simulink model "check_serial_2msg_processor_2"  (R2021a)
settings: Solver=FixedStepDiscrete  StartTime=0.0  StopTime=inf  FixedStep=time_step  RelTol=1e-3
model workspace (MAT data in the model file):
  time_step = 0.01
undefined symbols (not defined in the file or in its folder): DiscIntNeverNeededParam, Serial_Port, Standard_Devices
libraries: sldrtlib x6
settings Model: OrderedModelArguments=off  Creator=Rahul Subramanian  LastModifiedBy=Rahul Subramanian
settings SolverCC: AlgebraicLoopSolver=TrustRegion
settings DebuggingCC: SFMachineParentedDataDiag=warning
settings RTWCC: Description=Simulink Desktop Real-Time  SystemTargetFile=sldrt.tlc  TemplateMakefile=sldrt.tmf  RTWCompilerOptimization=on
settings CodeAppCC: MaxIdLength=95
settings SimulinkDesktopRealTimeCC: TargetPreCompLibLocation=C:\Program Files\MATLAB\R2021a\toolbox\sldrt\lib\win64

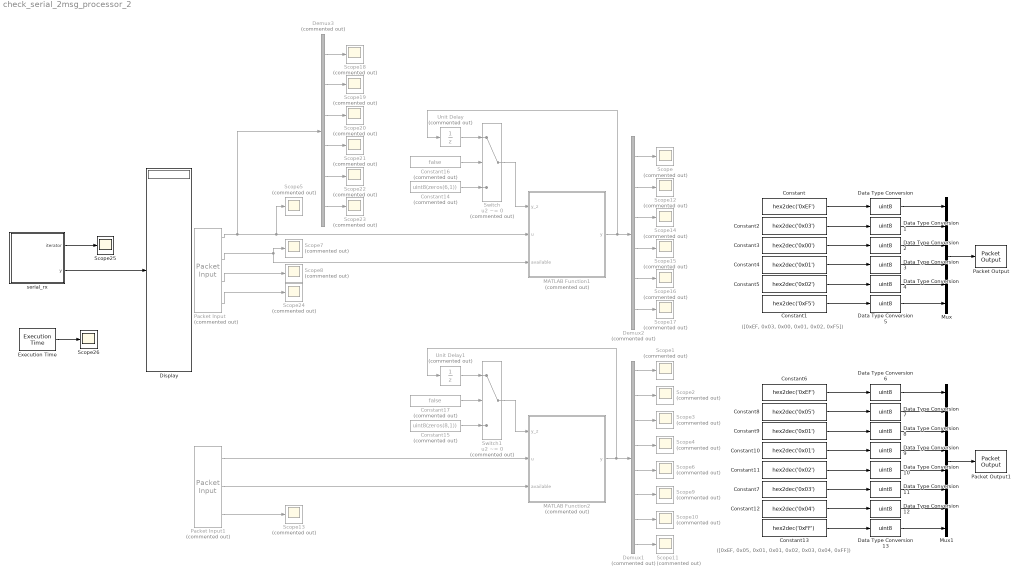
== system check_serial_2msg_processor_2 ==
  note: ([0xEF, 0x05, 0x01, 0x01, 0x02, 0x03, 0x04, 0xFF])
  note: ([0xEF, 0x03, 0x00, 0x01, 0x02, 0xF5])
  Constant : Constant  Value=hex2dec('0xEF')
  Constant1 : Constant  Value=hex2dec('0xF5')
  Constant10 : Constant  Value=hex2dec('0x01')
  Constant11 : Constant  Value=hex2dec('0x02')
  Constant12 : Constant  Value=hex2dec('0x04')
  Constant13 : Constant  Value=hex2dec('0xFF')
  Constant14 : Constant  Commented=on  Value=uint8(zeros(6,1))
  Constant15 : Constant  Commented=on  Value=uint8(zeros(8,1))
  Constant16 : Constant  Commented=on  Value=false
  Constant17 : Constant  Commented=on  Value=false
  Constant2 : Constant  Value=hex2dec('0x03')
  Constant3 : Constant  Value=hex2dec('0x00')
  Constant4 : Constant  Value=hex2dec('0x01')
  Constant5 : Constant  Value=hex2dec('0x02')
  Constant6 : Constant  Value=hex2dec('0xEF')
  Constant7 : Constant  Value=hex2dec('0x03')
  Constant8 : Constant  Value=hex2dec('0x05')
  Constant9 : Constant  Value=hex2dec('0x01')
  Data Type Conversion{,1..13} (14 alike) : DataTypeConversion  OutDataTypeStr=uint8
  Demux1 : Demux  Commented=on  Outputs=8
  Demux2 : Demux  Commented=on  Outputs=6
  Demux3 : Demux  Commented=on  Outputs=6
  Display : Display
  Execution Time : sldrtlib/Target Profiling/Execution Time  ShowTaskTimes=off
      settings: SourceProductBaseCode=WT
  MATLAB Function1 : MATLAB Function  Commented=on  TreatAsAtomicUnit=on
  MATLAB Function2 : MATLAB Function  Commented=on  TreatAsAtomicUnit=on
  Mux : Mux  Inputs=6
  Mux1 : Mux  Inputs=8
  Packet Input : sldrtlib/Packet Input  Commented=on  SampleTime=time_step  MaxMissedTicks=inf  ShowMissedTicks=on  YieldWhenWaiting=off  DrvName=Standard_Devices/Serial_Port  DrvAddress=5  DrvOptions=[115200 8 0 0 0 0 0 0]  PacketSize=6  DataTypes='6*uint8'  ShowReady=on  ShowError=on  PacketID=1  ByteOrder=1  ShowTimestamp=off
      settings: AttributesFormatString=Serial Port [5]
  Packet Input1 : sldrtlib/Packet Input  Commented=on  SampleTime=time_step  MaxMissedTicks=inf  ShowMissedTicks=on  YieldWhenWaiting=off  DrvName=Standard_Devices/Serial_Port  DrvAddress=5  DrvOptions=[115200 8 0 0 0 0 0 0]  PacketSize=8  DataTypes='8*uint8'  ShowReady=on  ShowError=off  PacketID=1  ByteOrder=1  ShowTimestamp=off
      settings: AttributesFormatString=Serial Port [5]
  Packet Output : sldrtlib/Packet Output  SampleTime=time_step  MaxMissedTicks=inf  ShowMissedTicks=off  YieldWhenWaiting=off  DrvName=Standard_Devices/Serial_Port  DrvAddress=5  DrvOptions=[115200 8 0 0 0 0 0 0]  PacketSize=6  DataTypes='6*uint8'  ShowReady=off  ShowError=off  PacketID=1  ByteOrder=1  InitialValue=[]  FinalValue=[]
      settings: AttributesFormatString=Serial Port [5]
  Packet Output1 : sldrtlib/Packet Output  SampleTime=time_step  MaxMissedTicks=inf  ShowMissedTicks=off  YieldWhenWaiting=off  DrvName=Standard_Devices/Serial_Port  DrvAddress=5  DrvOptions=[115200 8 0 0 0 0 0 0]  PacketSize=8  DataTypes='8*uint8'  ShowReady=off  ShowError=off  PacketID=1  ByteOrder=1  InitialValue=[]  FinalValue=[]
      settings: AttributesFormatString=Serial Port [5]
  Scope{,1..24} (25 alike) : Scope  Commented=on
  Scope25 : Scope
  Scope26 : Scope
  Switch : Switch  Commented=on  Criteria=u2 ~= 0
  Switch1 : Switch  Commented=on  Criteria=u2 ~= 0
  Unit Delay : UnitDelay  Commented=on  SampleTime=-1  HasFrameUpgradeWarning=on
  Unit Delay1 : UnitDelay  Commented=on  SampleTime=-1  HasFrameUpgradeWarning=on
  serial_rx : Subsystem
  wires:
  Constant/1 -> Data Type Conversion/1
  Constant2/1 -> Data Type Conversion1/1
  Constant3/1 -> Data Type Conversion2/1
  Constant4/1 -> Data Type Conversion3/1
  Constant5/1 -> Data Type Conversion4/1
  Data Type Conversion/1 -> Mux/1
  Data Type Conversion1/1 -> Mux/2
  Data Type Conversion2/1 -> Mux/3
  Data Type Conversion3/1 -> Mux/4
  Data Type Conversion4/1 -> Mux/5
  Packet Input/3 -> Scope8/1
  Mux/1 -> Packet Output/1
  Constant1/1 -> Data Type Conversion5/1
  Data Type Conversion5/1 -> Mux/6
  Data Type Conversion11/1 -> Mux1/6
  Constant7/1 -> Data Type Conversion11/1
  Mux1/1 -> Packet Output1/1
  Data Type Conversion10/1 -> Mux1/5
  Data Type Conversion9/1 -> Mux1/4
  Data Type Conversion8/1 -> Mux1/3
  Data Type Conversion7/1 -> Mux1/2
  Data Type Conversion6/1 -> Mux1/1
  Constant11/1 -> Data Type Conversion10/1
  Constant10/1 -> Data Type Conversion9/1
  Constant9/1 -> Data Type Conversion8/1
  Constant8/1 -> Data Type Conversion7/1
  Constant6/1 -> Data Type Conversion6/1
  Data Type Conversion12/1 -> Mux1/7
  Data Type Conversion13/1 -> Mux1/8
  Constant12/1 -> Data Type Conversion12/1
  Constant13/1 -> Data Type Conversion13/1
  Demux2/1 -> Scope/1
  MATLAB Function1/1(y) -> Unit Delay/1, Demux2/1
  Demux2/2 -> Scope12/1
  Demux2/3 -> Scope14/1
  Demux2/4 -> Scope15/1
  Demux2/5 -> Scope16/1
  Demux2/6 -> Scope17/1
  Switch/1 -> MATLAB Function1/1(y_z)
  Demux1/6 -> Scope9/1
  Demux1/5 -> Scope6/1
  Demux1/4 -> Scope4/1
  Demux1/3 -> Scope3/1
  Demux1/2 -> Scope2/1
  MATLAB Function2/1(y) -> Unit Delay1/1, Demux1/1
  Demux1/1 -> Scope1/1
  Packet Input/2 -> MATLAB Function1/3(available), Scope7/1
  Demux1/8 -> Scope11/1
  Demux1/7 -> Scope10/1
  Packet Input1/1 -> MATLAB Function2/2(u)
  Packet Input1/2 -> MATLAB Function2/3(available)
  Unit Delay/1 -> Switch/1
  Constant16/1 -> Switch/2
  Constant14/1 -> Switch/3
  Constant15/1 -> Switch1/3
  Constant17/1 -> Switch1/2
  Unit Delay1/1 -> Switch1/1
  Switch1/1 -> MATLAB Function2/1(y_z)
  Packet Input1/3 -> Scope13/1
  Demux3/6 -> Scope23/1
  Demux3/5 -> Scope22/1
  Demux3/4 -> Scope21/1
  Demux3/3 -> Scope20/1
  Demux3/2 -> Scope19/1
  Packet Input/1 -> Demux3/1, MATLAB Function1/2(u), Scope5/1
  Demux3/1 -> Scope18/1
  Packet Input/4 -> Scope24/1
  Execution Time/1 -> Scope26/1
  serial_rx/1(iterator) -> Scope25/1
  serial_rx/2(y) -> Display/1

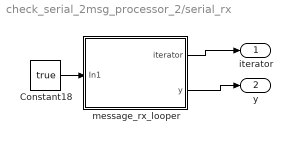
== system check_serial_2msg_processor_2/serial_rx ==
  Constant18 : Constant  Value=true
  message_rx_looper : Subsystem  TreatAsAtomicUnit=on
  iterator : Outport
  y : Outport  Port=2
  wires:
  Constant18/1 -> message_rx_looper/1(In1)
  message_rx_looper/2(y) -> y/1
  message_rx_looper/1(iterator) -> iterator/1

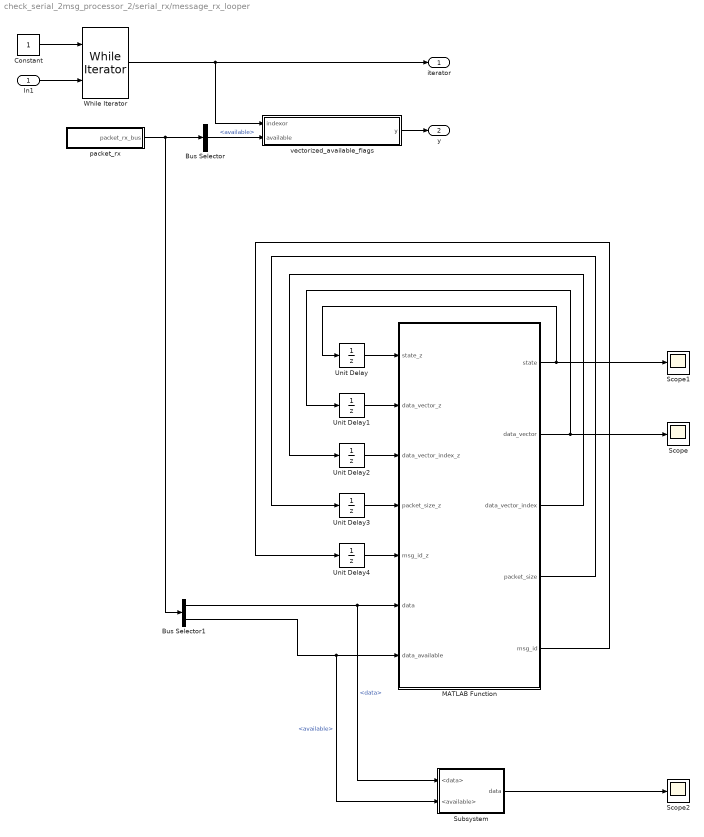
== system check_serial_2msg_processor_2/serial_rx/message_rx_looper ==
  In1 : Inport
  Bus Selector : BusSelector  OutputSignals=available
  Bus Selector1 : BusSelector  OutputSignals=data,available
  Constant : Constant
  MATLAB Function : MATLAB Function  TreatAsAtomicUnit=on
  Scope : Scope
  Scope1 : Scope
  Scope2 : Scope
  Subsystem : Subsystem
  Unit Delay{,1..4} (5 alike) : UnitDelay  SampleTime=-1  HasFrameUpgradeWarning=on
  While Iterator : WhileIterator  MaxIters=144  ResetStates=reset  ShowIterationPort=on  OutputDataType=uint8
  packet_rx : Subsystem
  vectorized_available_flags : Subsystem
  iterator : Outport
  y : Outport  Port=2
  wires:
  While Iterator/1 -> vectorized_available_flags/1(indexor), iterator/1
  In1/1 -> While Iterator/2
  vectorized_available_flags/1(y) -> y/1
  Constant/1 -> While Iterator/1
  packet_rx/1(packet_rx_bus) -> Bus Selector/1, Bus Selector1/1
  Bus Selector/1 -> vectorized_available_flags/2(available)  "<available>"
  Bus Selector1/1 -> Subsystem/1(<data>), MATLAB Function/6(data)  "<data>"
  Bus Selector1/2 -> Subsystem/2(<available>), MATLAB Function/7(data_available)  "<available>"
  Unit Delay/1 -> MATLAB Function/1(state_z)
  MATLAB Function/1(state) -> Scope1/1, Unit Delay/1
  MATLAB Function/2(data_vector) -> Scope/1, Unit Delay1/1
  Unit Delay1/1 -> MATLAB Function/2(data_vector_z)
  Unit Delay2/1 -> MATLAB Function/3(data_vector_index_z)
  MATLAB Function/3(data_vector_index) -> Unit Delay2/1
  Unit Delay3/1 -> MATLAB Function/4(packet_size_z)
  MATLAB Function/4(packet_size) -> Unit Delay3/1
  Unit Delay4/1 -> MATLAB Function/5(msg_id_z)
  MATLAB Function/5(msg_id) -> Unit Delay4/1
  Subsystem/1(data) -> Scope2/1

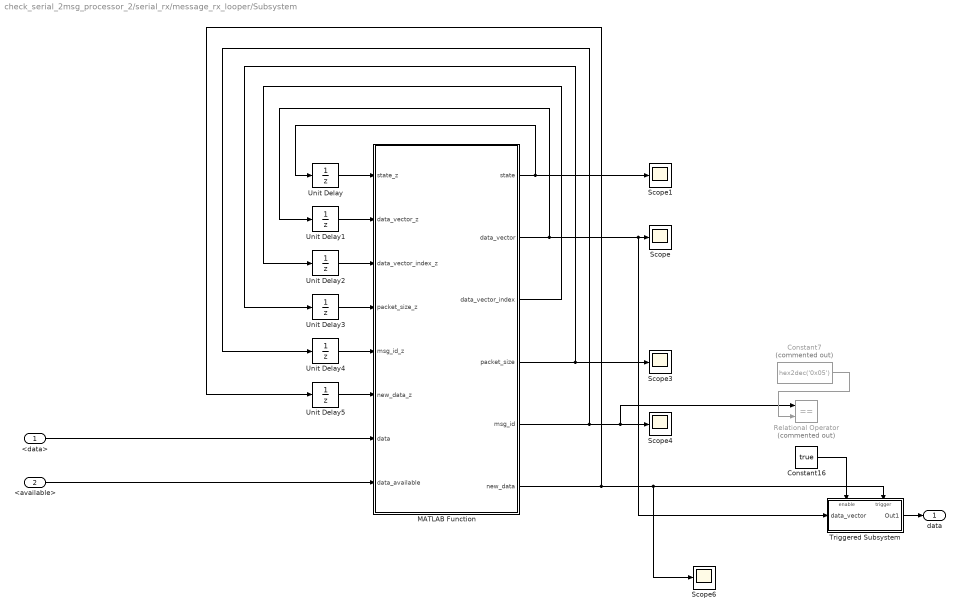
== system check_serial_2msg_processor_2/serial_rx/message_rx_looper/Subsystem ==
  <data> : Inport
  <available> : Inport  Port=2
  Constant16 : Constant  Value=true
  Constant7 : Constant  Commented=on  Value=hex2dec('0x05')
  MATLAB Function : MATLAB Function  TreatAsAtomicUnit=on
  Relational Operator : RelationalOperator  Commented=on  Operator===  OutDataTypeStr=boolean  RndMeth=Simplest
  Scope{,1,3..4,6} (5 alike) : Scope
  Triggered Subsystem : Subsystem  TreatAsAtomicUnit=on
  Unit Delay : UnitDelay  InitialCondition=uint8(1)  SampleTime=-1  HasFrameUpgradeWarning=on
  Unit Delay1 : UnitDelay  SampleTime=-1  HasFrameUpgradeWarning=on
  Unit Delay2 : UnitDelay  InitialCondition=1  SampleTime=-1  HasFrameUpgradeWarning=on
  Unit Delay3 : UnitDelay  SampleTime=-1  HasFrameUpgradeWarning=on
  Unit Delay4 : UnitDelay  SampleTime=-1  HasFrameUpgradeWarning=on
  Unit Delay5 : UnitDelay  InitialCondition=false  SampleTime=-1  HasFrameUpgradeWarning=on
  data : Outport
  wires:
  <data>/1 -> MATLAB Function/7(data)
  MATLAB Function/6(new_data) -> Unit Delay5/1, Scope6/1, Triggered Subsystem/Trigger
  Constant16/1 -> Triggered Subsystem/Enable
  MATLAB Function/1(state) -> Scope1/1, Unit Delay/1
  Unit Delay/1 -> MATLAB Function/1(state_z)
  Unit Delay3/1 -> MATLAB Function/4(packet_size_z)
  MATLAB Function/2(data_vector) -> Triggered Subsystem/1(data_vector), Scope/1, Unit Delay1/1
  Unit Delay1/1 -> MATLAB Function/2(data_vector_z)
  MATLAB Function/5(msg_id) -> Relational Operator/1, Scope4/1, Unit Delay4/1
  MATLAB Function/4(packet_size) -> Unit Delay3/1, Scope3/1
  MATLAB Function/3(data_vector_index) -> Unit Delay2/1
  Unit Delay2/1 -> MATLAB Function/3(data_vector_index_z)
  Unit Delay4/1 -> MATLAB Function/5(msg_id_z)
  Constant7/1 -> Relational Operator/2
  Unit Delay5/1 -> MATLAB Function/6(new_data_z)
  Triggered Subsystem/1(Out1) -> data/1
  <available>/1 -> MATLAB Function/8(data_available)

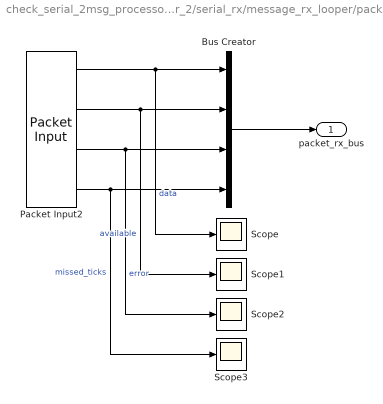
== system check_serial_2msg_processor_2/serial_rx/message_rx_looper/packet_rx ==
  Bus Creator : BusCreator  Inputs=4
  Packet Input2 : sldrtlib/Packet Input  SampleTime=-1  MaxMissedTicks=inf  ShowMissedTicks=on  YieldWhenWaiting=off  DrvName=Standard_Devices/Serial_Port  DrvAddress=5  DrvOptions=[115200 8 0 0 0 0 0 0]  PacketSize=1  DataTypes='1*uint8'  ShowReady=on  ShowError=on  PacketID=1  ByteOrder=1  ShowTimestamp=off
      settings: AttributesFormatString=Serial Port [5]
  Scope{,1..3} (4 alike) : Scope
  packet_rx_bus : Outport
  wires:
  Packet Input2/4 -> Bus Creator/4, Scope3/1  "missed_ticks"
  Packet Input2/1 -> Bus Creator/1, Scope/1  "data"
  Packet Input2/2 -> Bus Creator/2, Scope1/1  "available"
  Packet Input2/3 -> Bus Creator/3, Scope2/1  "error"
  Bus Creator/1 -> packet_rx_bus/1

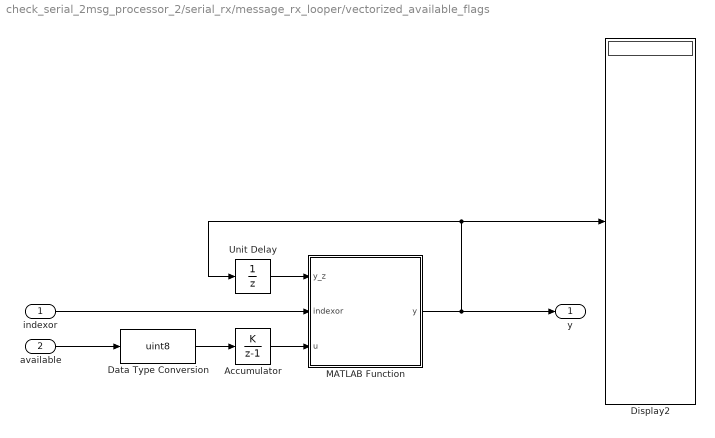
== system check_serial_2msg_processor_2/serial_rx/message_rx_looper/vectorized_available_flags ==
  indexor : Inport
  available : Inport  Port=2
  Accumulator : DiscreteIntegrator  IntegratorMethod=Accumulation: Forward Euler  SampleTime=-1  ICPrevOutput=DiscIntNeverNeededParam  ICPrevScaledInput=DiscIntNeverNeededParam
  Data Type Conversion : DataTypeConversion  OutDataTypeStr=uint8
  Display2 : Display
  MATLAB Function : MATLAB Function  TreatAsAtomicUnit=on
  Unit Delay : UnitDelay  SampleTime=-1  HasFrameUpgradeWarning=on
  y : Outport
  wires:
  Data Type Conversion/1 -> Accumulator/1
  MATLAB Function/1(y) -> y/1, Display2/1, Unit Delay/1
  Accumulator/1 -> MATLAB Function/3(u)
  Unit Delay/1 -> MATLAB Function/1(y_z)
  available/1 -> Data Type Conversion/1
  indexor/1 -> MATLAB Function/2(indexor)

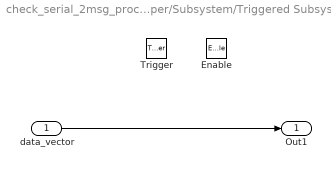
== system check_serial_2msg_processor_2/serial_rx/message_rx_looper/Subsystem/Triggered Subsystem ==
  data_vector : Inport
  Enable : EnablePort
  Trigger : TriggerPort  VariantControl=(inherit)
  Out1 : Outport
  wires:
  data_vector/1 -> Out1/1

== matlab function check_serial_2msg_processor_2/MATLAB Function1 ==
  data: y_z input size=6; u input uint8; y output uint8 size=6; available input
function y  = fcn(y_z, u, available)

y = y_z;
data_packet_size = uint8(0);

if available
    if u(1) == hex2dec('0xEF')
        if u(3) == 0
            for j = 1:6
                y(j) = u(j);
            end
    %             data_packet_size = u(2) - 1;
    %             data_id = u(3);
    %             data(1) = u(4);
    %             data(2) = u(5);
    %             crc(3) = u(6);
        end
    end
end

== matlab function check_serial_2msg_processor_2/MATLAB Function2 ==
  data: y_z input size=8; u input uint8; y output uint8 size=8; available input
function y  = fcn(y_z, u, available)

y = y_z;
data_packet_size = uint8(0);

if available
    if u(1) == hex2dec('0xEF')
        if u(3) == 1
            for j = 1:8
                y(j) = u(j);
            end
    %             data_packet_size = u(2) - 1;
    %             data_id = u(3);
    %             data(1) = u(4);
    %             data(2) = u(5);
    %             crc(3) = u(6);
        end
    end
end

== matlab function check_serial_2msg_processor_2/serial_rx/message_rx_looper/MATLAB Function ==
  data: state_z input uint8; data_vector_z input uint8 size=4; data_vector_index_z input uint8; packet_size_z input uint8; msg_id_z input uint8; data input uint8; state output uint8; data_available input boolean; data_vector output uint8 size=4; data_vector_index output uint8; packet_size output uint8; msg_id output uint8
function [state, data_vector, data_vector_index, packet_size, msg_id]    = fcn(state_z, data_vector_z, data_vector_index_z, packet_size_z, msg_id_z, data, data_available)

% read previous state
state = state_z;
data_vector = data_vector_z;
data_vector_index = data_vector_index_z;
packet_size = packet_size_z;
msg_id = msg_id_z;

switch state
    
    case uint8(1)
        if data_available
            if data == hex2dec('0xEF')
                state = uint8(2);
            end
        end

    case uint8(2)
        if data_available
            if data == hex2dec('0xEF')
                state = uint8(3);
            end
        end

    case uint8(3)
        if data_available
            packet_size = data - 1;
            state = uint8(4);
        end

    case uint8(4)
        if data_available
            msg_id = data;
            state = uint8(5);
        end

    case uint8(5)
        if data_available
            data_vector(data_vector_index) = data;
            data_vector_index = data_vector_index + 1;

            if data_vector_index == packet_size
                state = uint8(6);
            end
        end

	case uint8(6)
        if data_available
            crc = data;
%             if crc == func(crc)
            if crc ~= 0
                new_data = true; % call the function
                state = uint8(0);
                state = uint8(0);
                data_vector = uint8(zeros(4,1));
                data_vector_index = uint8(0);
                packet_size = uint8(0);
            end
        end
end

== matlab function check_serial_2msg_processor_2/serial_rx/message_rx_looper/vectorized_available_flags/MATLAB Function ==
  data: y_z input; indexor input; u input uint8; y output uint8 size=144
function y = fcn(y_z, indexor, u)

y = y_z;
y(indexor) = u;

== matlab function check_serial_2msg_processor_2/serial_rx/message_rx_looper/Subsystem/MATLAB Function ==
  data: state_z input uint8; data_vector_z input uint8 size=4; data_vector_index_z input uint8; packet_size_z input uint8; msg_id_z input uint8; new_data_z input boolean; data input uint8; state output uint8; data_available input boolean; data_vector output uint8 size=4; data_vector_index output uint8; packet_size output uint8; msg_id output uint8; new_data output boolean
function [state, data_vector, data_vector_index, packet_size, msg_id, new_data] = fcn(state_z, data_vector_z, data_vector_index_z, packet_size_z, msg_id_z, new_data_z, data, data_available)

% read previous state
state = state_z;
data_vector = data_vector_z;
data_vector_index = data_vector_index_z;
packet_size = packet_size_z;
msg_id = msg_id_z;
new_data = new_data_z;

switch state
    
    case uint8(1)
        if data_available
            if data == hex2dec('0xEF')
                state = state + 1;
                new_data = false;
                msg_id = uint8(0);
                data_vector = uint8(zeros(4,1));
                data_vector_index = uint8(1);
                packet_size = uint8(0);
            end
        end

    case uint8(2)
        if data_available
            packet_size = data - 1;
            state = state + 1;
        end

    case uint8(3)
        if data_available
            msg_id = data;
            state = state + 1;
        end

    case uint8(4)
        if data_available
            data_vector(data_vector_index) = data;
            
            if data_vector_index == packet_size
                state = state + 1;
            end
            
            data_vector_index = data_vector_index + 1;

        end

	case uint8(5)
        if data_available
            crc = data;
%             if crc == func(crc)
            if crc ~= 0
                new_data = true; % call the function
                state = uint8(1);
                
            end
        end
end
